simulink model "Impedance_Jawwad"  (R2023a)
settings: Solver=VariableStepAuto  StartTime=0.0  StopTime=10.0  RelTol=1e-3
values from neighbouring files (symbols this model uses):
  Kd = diag([50,50,50,50,50,50])    [parameters.m]
  Kp = diag([250,250,250,250,250,250])    [parameters.m]
  Md = diag([3,3,3,3,3,3])    [parameters.m]
undefined symbols (not defined in the file or in its folder): parms
libraries: robotcorelib x1
settings Model: Creator=uzair  LastModifiedBy=syedj
settings OptimizationCC: ReuseModelBlockBuffer=off

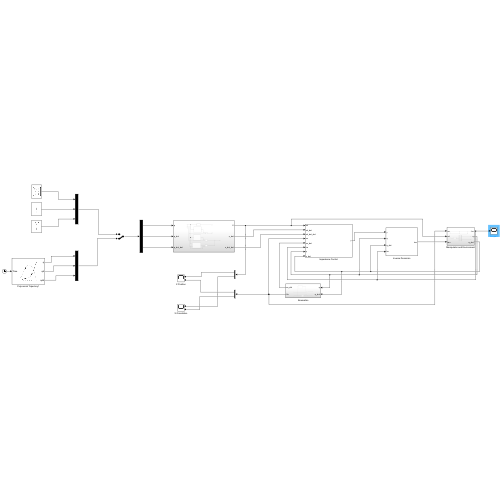
[thumbnail: Simulink's stored preview of the top-level diagram]
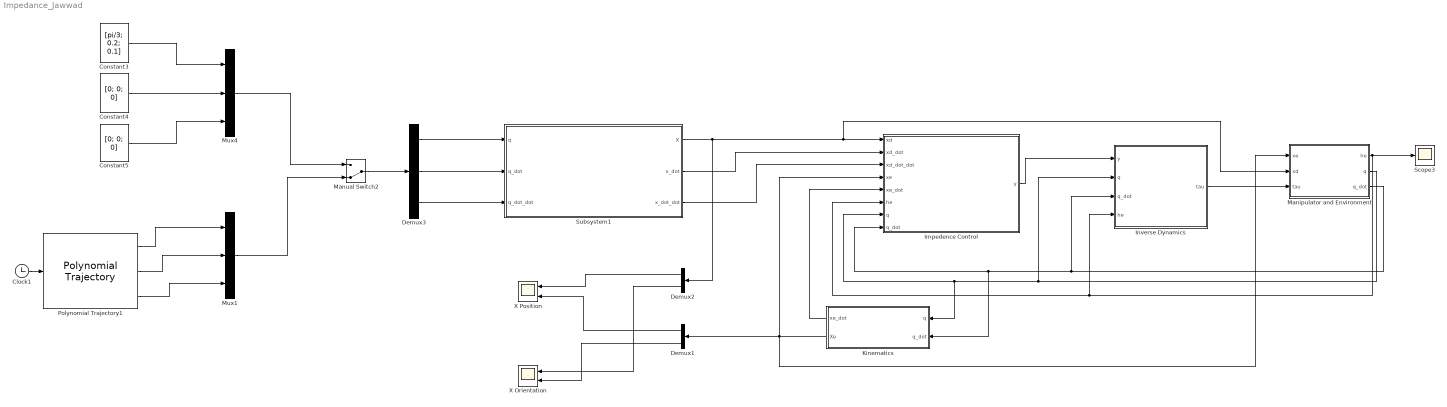
== system Impedance_Jawwad ==
  Clock1 : Clock
  Constant3 : Constant  Value=[pi/3; 0.2; 0.1]  VectorParams1D=off
  Constant4 : Constant  Value=[0; 0; 0]  VectorParams1D=off
  Constant5 : Constant  Value=[0; 0; 0]  VectorParams1D=off
  Demux1 : Demux  Outputs=2
  Demux2 : Demux  Outputs=2
  Demux3 : Demux  Outputs=3
  Impedence Control : Subsystem
  Inverse Dynamics : Subsystem
  Kinematics : Subsystem
  Manipulator and Environment : Subsystem
  Manual Switch2 : ManualSwitch  CurrentSetting=0
  Mux1 : Mux  Inputs=3
  Mux4 : Mux  Inputs=3
  Polynomial Trajectory1 : robotcorelib/Polynomial Trajectory  WaypointSource=Internal  Waypoints=[ 0,0.5,0.7,0.9; 0,-0.05,-0.1,-0.1; 0,0.5,0.7,0.9]  TimePoints=[ 0, 4, 7, 10]  TimeInterval=[ 1, 4 ]  Method=Cubic Polynomial  ParameterSource=Internal  VelocityBoundaryCondition=zeros( 3,4 )  AccelerationBoundaryCondition=zeros( 3,4 )  SimulateUsing=Interpreted execution
  Scope3 : Scope
  Subsystem1 : Subsystem
  X Orientation : Scope  NumInputPorts=2
  X Position : Scope  NumInputPorts=2
  wires:
  Demux1/2 -> X Orientation/2
  Demux2/2 -> X Orientation/1
  Demux2/1 -> X Position/1
  Demux1/1 -> X Position/2
  Manual Switch2/1 -> Demux3/1
  Mux4/1 -> Manual Switch2/1
  Constant4/1 -> Mux4/2
  Polynomial Trajectory1/1 -> Mux1/1
  Polynomial Trajectory1/3 -> Mux1/3
  Mux1/1 -> Manual Switch2/2
  Constant5/1 -> Mux4/3
  Clock1/1 -> Polynomial Trajectory1/1
  Constant3/1 -> Mux4/1
  Demux3/3 -> Subsystem1/3(q_dot_dot)
  Polynomial Trajectory1/2 -> Mux1/2
  Demux3/2 -> Subsystem1/2(q_dot)
  Impedence Control/1(y) -> Inverse Dynamics/1(y)
  Subsystem1/1(X) -> Demux2/1, Manipulator and Environment/2(xd), Impedence Control/1(xd)
  Subsystem1/2(x_dot) -> Impedence Control/2(xd_dot)
  Subsystem1/3(x_dot_dot) -> Impedence Control/3(xd_dot_dot)
  Kinematics/2(Xe) -> Manipulator and Environment/1(xe), Demux1/1, Impedence Control/4(xe)
  Kinematics/1(xe_dot) -> Impedence Control/5(xe_dot)
  Manipulator and Environment/2(q) -> Inverse Dynamics/2(q), Kinematics/1(q), Impedence Control/7(q)
  Manipulator and Environment/3(q_dot) -> Inverse Dynamics/3(q_dot), Kinematics/2(q_dot), Impedence Control/8(q_dot)
  Manipulator and Environment/1(he) -> Scope3/1, Inverse Dynamics/4(he), Impedence Control/6(he)
  Inverse Dynamics/1(tau) -> Manipulator and Environment/3(tau)
  Demux3/1 -> Subsystem1/1(q)

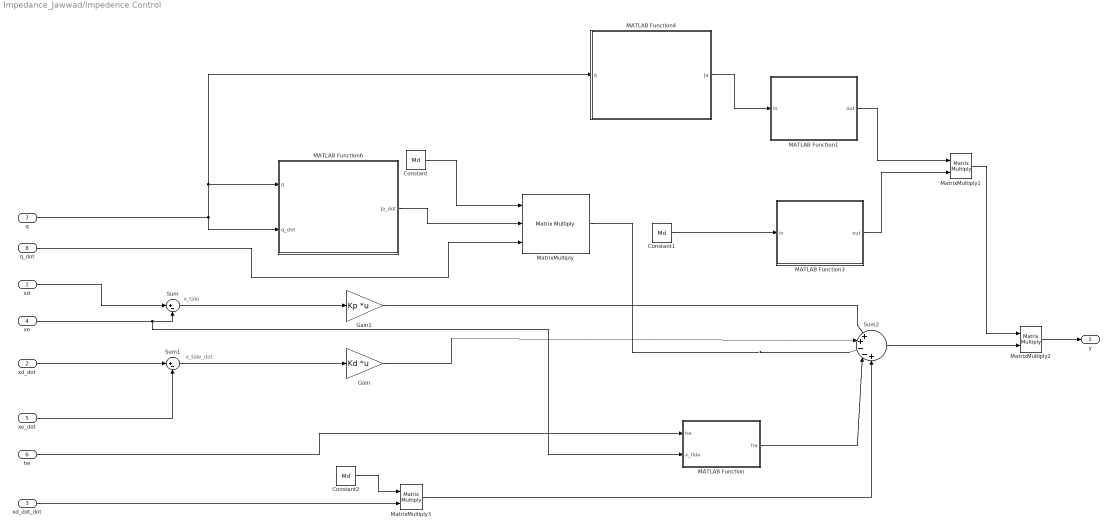
== system Impedance_Jawwad/Impedence Control ==
  note: x_tide_dot
  note: x_tide
  xd : Inport
  xd_dot : Inport  Port=2
  xd_dot_dot : Inport  Port=3
  xe : Inport  Port=4
  xe_dot : Inport  Port=5
  he : Inport  Port=6
  q : Inport  Port=7
  q_dot : Inport  Port=8
  Constant : Constant  Value=Md  VectorParams1D=off
  Constant1 : Constant  Value=Md  VectorParams1D=off
  Constant2 : Constant  Value=Md
  Gain : Gain  Gain=Kd  Multiplication=Matrix(K*u)
  Gain1 : Gain  Gain=Kp  Multiplication=Matrix(K*u)
  MATLAB Function : MATLAB Function  TreatAsAtomicUnit=on
  MATLAB Function1 : MATLAB Function  TreatAsAtomicUnit=on
  MATLAB Function3 : MATLAB Function  TreatAsAtomicUnit=on
  MATLAB Function4 : MATLAB Function  TreatAsAtomicUnit=on
  MATLAB Function6 : MATLAB Function  TreatAsAtomicUnit=on
  MatrixMultiply : Product  Inputs=3  Multiplication=Matrix(*)
  MatrixMultiply1 : Product  Multiplication=Matrix(*)
  MatrixMultiply2 : Product  Multiplication=Matrix(*)
  MatrixMultiply3 : Product  Multiplication=Matrix(*)
  Sum : Sum  Inputs=|+-
  Sum1 : Sum  Inputs=|+-
  Sum2 : Sum  Inputs=|++--+
  y : Outport
  wires:
  xd/1 -> Sum/1
  xe/1 -> MATLAB Function/2(x_tide), Sum/2
  Sum/1 -> Gain1/1
  xd_dot/1 -> Sum1/1
  xe_dot/1 -> Sum1/2
  Sum1/1 -> Gain/1
  Gain1/1 -> Sum2/1
  Gain/1 -> Sum2/2
  q/1 -> MATLAB Function6/2(q_dot), MATLAB Function4/1(q), MATLAB Function6/1(q)
  q_dot/1 -> MatrixMultiply/3
  Constant/1 -> MatrixMultiply/1
  MATLAB Function6/1(Ja_dot) -> MatrixMultiply/2
  MatrixMultiply/1 -> Sum2/3
  he/1 -> MATLAB Function/1(he)
  MATLAB Function/1(ha) -> Sum2/4
  MATLAB Function1/1(out) -> MatrixMultiply1/1
  MATLAB Function3/1(out) -> MatrixMultiply1/2
  MATLAB Function4/1(Ja) -> MATLAB Function1/1(in)
  Constant1/1 -> MATLAB Function3/1(in)
  Sum2/1 -> MatrixMultiply2/2
  MatrixMultiply1/1 -> MatrixMultiply2/1
  MatrixMultiply2/1 -> y/1
  xd_dot_dot/1 -> MatrixMultiply3/2
  Constant2/1 -> MatrixMultiply3/1
  MatrixMultiply3/1 -> Sum2/5

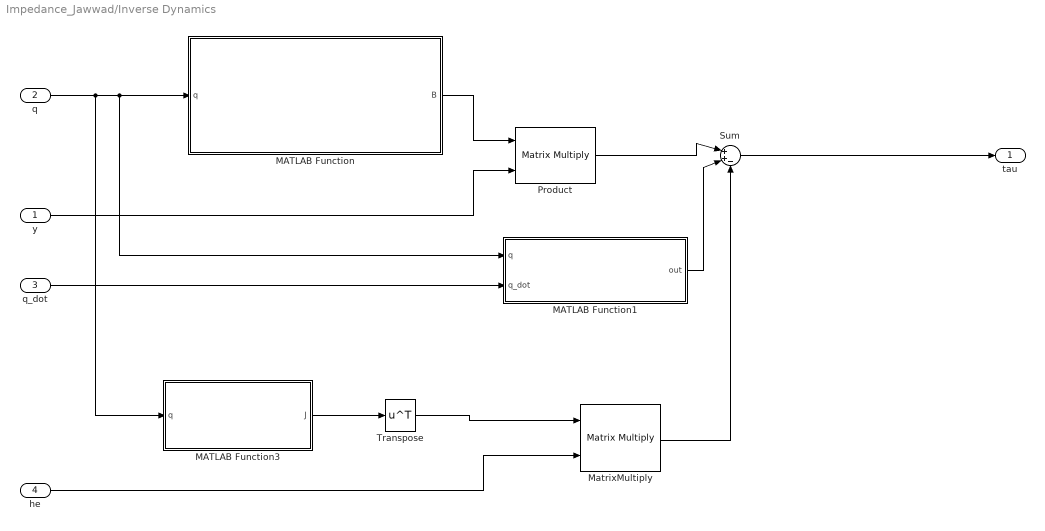
== system Impedance_Jawwad/Inverse Dynamics ==
  y : Inport
  q : Inport  Port=2
  q_dot : Inport  Port=3
  he : Inport  Port=4
  MATLAB Function : MATLAB Function  TreatAsAtomicUnit=on
  MATLAB Function1 : MATLAB Function  TreatAsAtomicUnit=on
  MATLAB Function3 : MATLAB Function  TreatAsAtomicUnit=on
  MatrixMultiply : Product  Multiplication=Matrix(*)
  Product : Product  Multiplication=Matrix(*)
  Sum : Sum  Inputs=|++-
  Transpose : Math  Operator=transpose  OutputSignalType=real
  tau : Outport
  wires:
  q/1 -> MATLAB Function3/1(q), MATLAB Function1/1(q), MATLAB Function/1(q)
  MATLAB Function/1(B) -> Product/1
  y/1 -> Product/2
  q_dot/1 -> MATLAB Function1/2(q_dot)
  MATLAB Function1/1(out) -> Sum/2
  Sum/1 -> tau/1
  MATLAB Function3/1(J) -> Transpose/1
  he/1 -> MatrixMultiply/2
  Transpose/1 -> MatrixMultiply/1
  MatrixMultiply/1 -> Sum/3
  Product/1 -> Sum/1

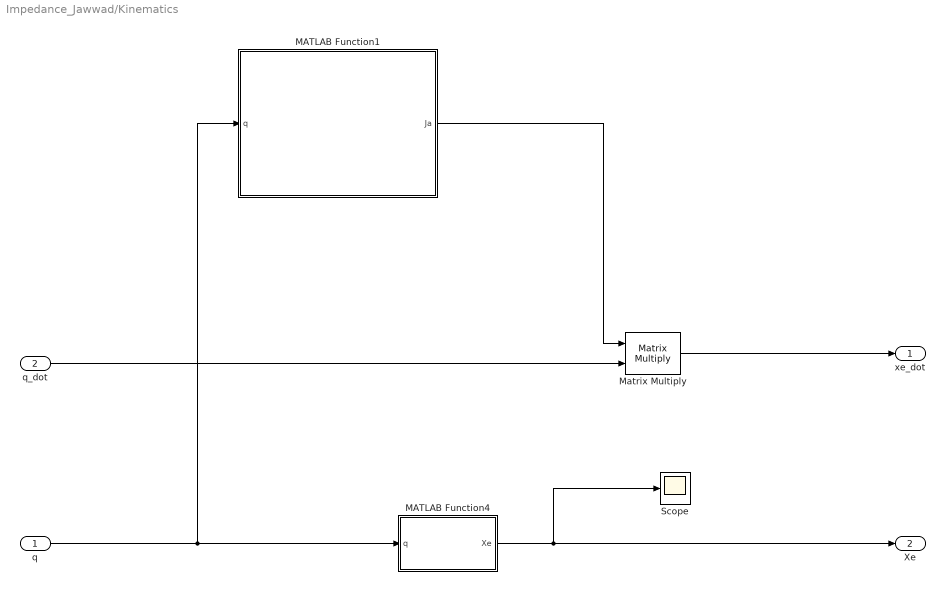
== system Impedance_Jawwad/Kinematics ==
  q : Inport
  q_dot : Inport  Port=2
  MATLAB Function1 : MATLAB Function  TreatAsAtomicUnit=on
  MATLAB Function4 : MATLAB Function  TreatAsAtomicUnit=on
  Matrix Multiply : Product  Multiplication=Matrix(*)
  Scope : Scope
  xe_dot : Outport
  Xe : Outport  Port=2
  wires:
  MATLAB Function1/1(Ja) -> Matrix Multiply/1
  q/1 -> MATLAB Function1/1(q), MATLAB Function4/1(q)
  MATLAB Function4/1(Xe) -> Scope/1, Xe/1
  Matrix Multiply/1 -> xe_dot/1
  q_dot/1 -> Matrix Multiply/2

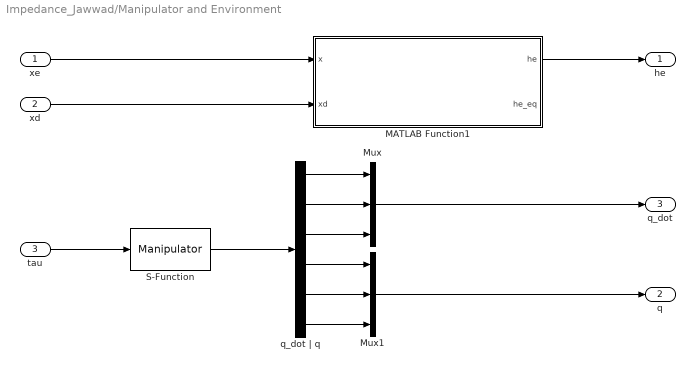
== system Impedance_Jawwad/Manipulator and Environment ==
  xe : Inport
  xd : Inport  Port=2
  tau : Inport  Port=3
  MATLAB Function1 : MATLAB Function  TreatAsAtomicUnit=on
  Mux : Mux  Inputs=3
  Mux1 : Mux  Inputs=3
  S-Function : S-Function  FunctionName=Manipulator  Parameters=params  SFunctionDeploymentMode=off  EnableBusSupport=off
  q_dot | q : Demux  Outputs=6
  he : Outport
  q : Outport  Port=2
  q_dot : Outport  Port=3
  wires:
  xe/1 -> MATLAB Function1/1(x)
  xd/1 -> MATLAB Function1/2(xd)
  MATLAB Function1/1(he) -> he/1
  S-Function/1 -> q_dot | q/1
  q_dot | q/4 -> Mux1/1
  q_dot | q/1 -> Mux/1
  q_dot | q/6 -> Mux1/3
  q_dot | q/2 -> Mux/2
  q_dot | q/5 -> Mux1/2
  q_dot | q/3 -> Mux/3
  Mux/1 -> q_dot/1
  Mux1/1 -> q/1
  tau/1 -> S-Function/1

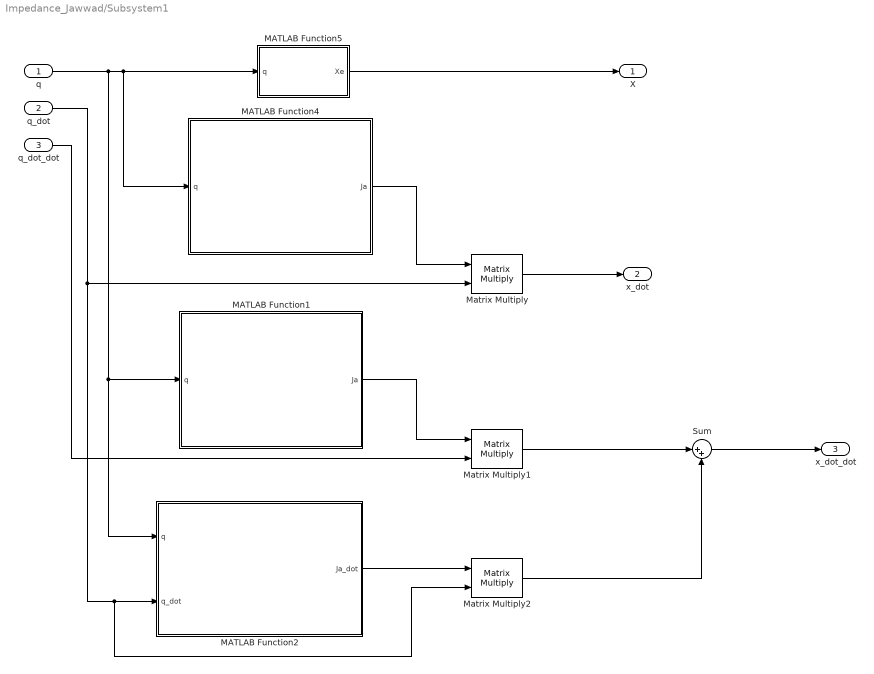
== system Impedance_Jawwad/Subsystem1 ==
  q : Inport
  q_dot : Inport  Port=2
  q_dot_dot : Inport  Port=3
  MATLAB Function1 : MATLAB Function  TreatAsAtomicUnit=on
  MATLAB Function2 : MATLAB Function  TreatAsAtomicUnit=on
  MATLAB Function4 : MATLAB Function  TreatAsAtomicUnit=on
  MATLAB Function5 : MATLAB Function  TreatAsAtomicUnit=on
  Matrix Multiply : Product  Multiplication=Matrix(*)
  Matrix Multiply1 : Product  Multiplication=Matrix(*)  SaturateOnIntegerOverflow=on  LockScale=on
  Matrix Multiply2 : Product  Multiplication=Matrix(*)  InputSameDT=on  SaturateOnIntegerOverflow=on
  Sum : Sum  Inputs=|++
  X : Outport
  x_dot : Outport  Port=2
  x_dot_dot : Outport  Port=3
  wires:
  q/1 -> MATLAB Function2/1(q), MATLAB Function1/1(q), MATLAB Function4/1(q), MATLAB Function5/1(q)
  MATLAB Function5/1(Xe) -> X/1
  Matrix Multiply/1 -> x_dot/1
  q_dot/1 -> MATLAB Function2/2(q_dot), Matrix Multiply2/2, Matrix Multiply/2
  MATLAB Function4/1(Ja) -> Matrix Multiply/1
  MATLAB Function1/1(Ja) -> Matrix Multiply1/1
  q_dot_dot/1 -> Matrix Multiply1/2
  Matrix Multiply1/1 -> Sum/1
  Sum/1 -> x_dot_dot/1
  MATLAB Function2/1(Ja_dot) -> Matrix Multiply2/1
  Matrix Multiply2/1 -> Sum/2

== matlab function Impedance_Jawwad/Impedence Control/MATLAB Function6 ==
  data: q input; Ja_dot output; q_dot input
function Ja_dot = AnalyticalJacobian_Dot(q, q_dot)
q1 = q(1);
q2 = q(2);
q3 = q(3);

q1_dot = q_dot(1);
q2_dot = q_dot(2);
q3_dot = q_dot(3);

    r1 = 0.4;
    a1 = 0.02;
    a2 = 0.03;
    a3 = 0.01;
    b1 = 0.1256;
    b2 = 0.03;
    b3 = 0.01;
    c1 = 0.4;
    c2 = 0.46;
    c3 = 0.15;

     H = [[0, -sin(q1), cos(q1),              cos(q1)*(c1 + c3 + q3)]
[1,        0,       0,                           - c2 - q2]
[0,  cos(q1), sin(q1), r1 + sin(q1)*(c3 + q3) + c1*sin(q1)]
[0,        0,       0,                                   1]];



eulers = rotm2eul(H(1:3,1:3), "ZYZ");


phi1 = eulers(1);
phi2 = eulers(2);
phi3 = eulers(3); %not used

Ja_dot_m = [
[        -cos(q1)*q1_dot*(c1 + c3 + q3)-sin(q1)*q3_dot,  0, -sin(q1)*q1_dot]
[                              0, 0,       0]
[         -sin(q1)*q1_dot*(c1 + c3 + q3)+cos(q1)*q3_dot,  0, cos(q1)*q1_dot]
[(cos(phi2)*sin(phi1))/sin(phi2),  0,       0]
[                     -cos(phi1),  0,       0]
[           -sin(phi1)/sin(phi2),  0,       0]
];

Ja_dot = Ja_dot_m;
end

== matlab function Impedance_Jawwad/Subsystem1/MATLAB Function2 ==
  data: q input; Ja_dot output; q_dot input
function Ja_dot = AnalyticalJacobian_Dot(q, q_dot)
q1 = q(1);
q2 = q(2);
q3 = q(3);

q1_dot = q_dot(1);
q2_dot = q_dot(2);
q3_dot = q_dot(3);

    r1 = 0.4;
    a1 = 0.02;
    a2 = 0.03;
    a3 = 0.01;
    b1 = 0.1256;
    b2 = 0.03;
    b3 = 0.01;
    c1 = 0.4;
    c2 = 0.46;
    c3 = 0.15;

    H = [[0, -sin(q1), cos(q1),              cos(q1)*(c1 + c3 + q3)]
[1,        0,       0,                           - c2 - q2]
[0,  cos(q1), sin(q1), r1 + sin(q1)*(c3 + q3) + c1*sin(q1)]
[0,        0,       0,                                   1]];



eulers = rotm2eul(H(1:3,1:3), "ZYZ");


phi1 = eulers(1);
phi2 = eulers(2);
phi3 = eulers(3); %not used

Ja_dot_m = [
[        -cos(q1)*q1_dot*(c1 + c3 + q3)-sin(q1)*q3_dot,  0, -sin(q1)*q1_dot]
[                              0, 0,       0]
[         -sin(q1)*q1_dot*(c1 + c3 + q3)+cos(q1)*q3_dot,  0, cos(q1)*q1_dot]
[(cos(phi2)*sin(phi1))/sin(phi2),  0,       0]
[                     -cos(phi1),  0,       0]
[           -sin(phi1)/sin(phi2),  0,       0]
];

Ja_dot = Ja_dot_m;
end

== matlab function Impedance_Jawwad/Subsystem1/MATLAB Function4 ==
  data: q input; Ja output
function Ja = AnalyticalJacobian(q)
    q1 = q(1);
    q2 = q(2);
    q3 = q(3);

    r1 = 0.4;
    a1 = 0.02;
    a2 = 0.03;
    a3 = 0.01;
    b1 = 0.1256;
    b2 = 0.03;
    b3 = 0.01;
    c1 = 0.4;
    c2 = 0.46;
    c3 = 0.15;

    H = [[0, -sin(q1), cos(q1),              cos(q1)*(c1 + c3 + q3)]
[1,        0,       0,                           - c2 - q2]
[0,  cos(q1), sin(q1), r1 + sin(q1)*(c3 + q3) + c1*sin(q1)]
[0,        0,       0,                                   1]];


eulers = rotm2eul(H(1:3,1:3), "ZYZ");


    phi1 = eulers(1);
    phi2 = eulers(2);
    phi3 = eulers(3); %not used

Ja_m = [
[        -sin(q1)*(c1 + c3 + q3),  0, cos(q1)]
[                              0, -1,       0]
[         cos(q1)*(c1 + c3 + q3),  0, sin(q1)]
[(cos(phi2)*sin(phi1))/sin(phi2),  0,       0]
[                     -cos(phi1),  0,       0]
[           -sin(phi1)/sin(phi2),  0,       0]
];


    Ja = Ja_m;
end

== matlab function Impedance_Jawwad/Subsystem1/MATLAB Function5 ==
  data: q input; Xe output
function Xe = Kinematics(q)
    q1 = q(1);
    q2 = q(2);
    q3 = q(3);

    r1 = 0.4;
    a1 = 0.02;
    a2 = 0.03;
    a3 = 0.01;
    b1 = 0.1256;
    b2 = 0.03;
    b3 = 0.01;
    c1 = 0.4;
    c2 = 0.46;
    c3 = 0.15;

    H = [[0, -sin(q1), cos(q1),              cos(q1)*(c1 + c3 + q3)]
[1,        0,       0,                           - c2 - q2]
[0,  cos(q1), sin(q1), r1 + sin(q1)*(c3 + q3) + c1*sin(q1)]
[0,        0,       0,                                   1]];

    eulers = rotm2eul(H(1:3,1:3), "ZYZ");

    Xe = [H(1:3,4); eulers'];
end

== matlab function Impedance_Jawwad/Inverse Dynamics/MATLAB Function1 ==
  data: q input; out output; q_dot input; params parameter
function out = n(q, q_dot, params)
    
    m1 = params.m(1);
    m2 = params.m(2);
    m3 = params.m(3);

    q1 = q(1);
    q2 = q(2);
    q3 = q(3);

    q1_dot = q_dot(1);
    q2_dot = q_dot(2);
    q3_dot = q_dot(3);
    
    r1 = 0.4;
    a1 = 0.02;
    a2 = 0.03;
    a3 = 0.01;
    b1 = 0.1256;
    b2 = 0.03;
    b3 = 0.01;
    c1 = 0.4;
    c2 = 0.46;
    c3 = 0.15;
    g = params.g;

    Fv = params.Fv;
 

   C = [[ (m3*q3_dot*(2*c1 + c3 + 2*q3))/2, 0, (m3*q1_dot*(2*c1 + c3 + 2*q3))/2]
[                                0, 0,                                0]
[-(m3*q1_dot*(2*c1 + c3 + 2*q3))/2, 0,                                0]];
   

G = [(c1*g*m1*cos(q1))/2 + g*m2*cos(q1)*(c1 - c2/2) + g*m3*cos(q1)*(c1 + c3/2 + q3)
        0;
        g*m3*sin(q1)];

    out = C*q_dot + diag(Fv)*q_dot + G;
end

== matlab function Impedance_Jawwad/Inverse Dynamics/MATLAB Function ==
  data: q input; B output; params parameter
function B = inertiaMatrix(q, params)
    q1 = q(1); % not used in this matrix
    q2 = q(2);
    q3 = q(3);

    m1 = params.m(1);
    m2 = params.m(2);
    m3 = params.m(3);
        
    r1 = 0.4;
    a1 = 0.02;
    a2 = 0.03;
    a3 = 0.01;
    b1 = 0.1256;
    b2 = 0.03;
    b3 = 0.01;
    c1 = 0.4;
    c2 = 0.46;
    c3 = 0.15;

  B = [[(a2^2*m2)/12 + (3*a1^4*m1)/2 + (a3^2*m3)/12 + (3*b1^4*m1)/2 + (b3^2*m3)/12 + c1^2*m1 + c1^2*m2 + c1^2*m3 + (7*c2^2*m2)/12 + (c3^2*m3)/2 + m3*q3^2 + 3*a1^2*b1^2*m1 - c1*c2*m2 + c1*c3*m3 + 2*c1*m3*q3 + c3*m3*q3,       0,  0]
[                                                                                                                                                                                                               0, m2 + m3,  0]
[                                                                                                                                                                                                               0,       0, m3]];
 end

== matlab function Impedance_Jawwad/Subsystem1/MATLAB Function1 ==
  data: q input; Ja output
function Ja = AnalyticalJacobian(q)
    q1 = q(1);
    q2 = q(2);
    q3 = q(3);

    r1 = 0.4;
    a1 = 0.02;
    a2 = 0.03;
    a3 = 0.01;
    b1 = 0.1256;
    b2 = 0.03;
    b3 = 0.01;
    c1 = 0.4;
    c2 = 0.46;
    c3 = 0.15;

    H = [[0, -sin(q1), cos(q1),              cos(q1)*(c1 + c3 + q3)]
[1,        0,       0,                           - c2 - q2]
[0,  cos(q1), sin(q1), r1 + sin(q1)*(c3 + q3) + c1*sin(q1)]
[0,        0,       0,                                   1]];


eulers = rotm2eul(H(1:3,1:3), "ZYZ");


    phi1 = eulers(1);
    phi2 = eulers(2);
    phi3 = eulers(3); %not used

Ja_m = [
[        -sin(q1)*(c1 + c3 + q3),  0, cos(q1)]
[                              0, -1,       0]
[         cos(q1)*(c1 + c3 + q3),  0, sin(q1)]
[(cos(phi2)*sin(phi1))/sin(phi2),  0,       0]
[                     -cos(phi1),  0,       0]
[           -sin(phi1)/sin(phi2),  0,       0]
];


    Ja = Ja_m;
end

== matlab function Impedance_Jawwad/Impedence Control/MATLAB Function ==
  data: he input; ha output; x_tide input
function ha = he_d_e(he, x_tide)

        euler = x_tide(4:6);

        phi1 = euler(1);
        phi2 = euler(2);

        T = [[0, -sin(phi1) ,    cos(phi1)*sin(phi2)];
                 [0,  cos(phi1) ,   sin(phi1)*sin(phi2)];
                 [1,               0  ,    cos(phi2)]];

        Ta = [[eye(3), zeros(3)];
              [zeros(3), T]];


        ha = Ta'*he;
end

== matlab function Impedance_Jawwad/Kinematics/MATLAB Function4 ==
  data: q input; Xe output
function Xe = Kinematics(q)
    q1 = q(1);
    q2 = q(2);
    q3 = q(3);
    
    r1 = 0.4;
    a1 = 0.02;
    a2 = 0.03;
    a3 = 0.01;
    b1 = 0.1256;
    b2 = 0.03;
    b3 = 0.01;
    c1 = 0.4;
    c2 = 0.46;
    c3 = 0.15;


    H = [[0, -sin(q1), cos(q1),              cos(q1)*(c1 + c3 + q3)]
[1,        0,       0,                           - c2 - q2]
[0,  cos(q1), sin(q1), r1 + sin(q1)*(c3 + q3) + c1*sin(q1)]
[0,        0,       0,                                   1]];
    
    eulers = rotm2eul(H(1:3,1:3), "ZYZ");

    Xe = [H(1:3,4); eulers'];
end

== matlab function Impedance_Jawwad/Impedence Control/MATLAB Function1 ==
  data: in input; out output
function out = inv(in)
    out = pinv(in);
end

== matlab function Impedance_Jawwad/Kinematics/MATLAB Function1 ==
  data: q input; Ja output
function Ja = AnalyticalJacobian(q)
    q1 = q(1);
    q2 = q(2);
    q3 = q(3);
    
    r1 = 0.4;
    a1 = 0.02;
    a2 = 0.03;
    a3 = 0.01;
    b1 = 0.1256;
    b2 = 0.03;
    b3 = 0.01;
    c1 = 0.4;
    c2 = 0.46;
    c3 = 0.15;

    H = [[0, -sin(q1), cos(q1),              cos(q1)*(c1 + c3 + q3)]
[1,        0,       0,                           - c2 - q2]
[0,  cos(q1), sin(q1), r1 + sin(q1)*(c3 + q3) + c1*sin(q1)]
[0,        0,       0,                                   1]];


eulers = rotm2eul(H(1:3,1:3), "ZYZ");


    phi1 = eulers(1);
    phi2 = eulers(2);
    phi3 = eulers(3); %not used

Ja_m = [
[        -sin(q1)*(c1 + c3 + q3),  0, cos(q1)]
[                              0, -1,       0]
[         cos(q1)*(c1 + c3 + q3),  0, sin(q1)]
[(cos(phi2)*sin(phi1))/sin(phi2),  0,       0]
[                     -cos(phi1),  0,       0]
[           -sin(phi1)/sin(phi2),  0,       0]
];


    Ja = Ja_m;
end

== matlab function Impedance_Jawwad/Manipulator and Environment/MATLAB Function1 ==
  data: x input; he output; xd input; parms parameter; Kp parameter; he_eq output
function [he,he_eq]= Environment(x, xd, parms, Kp)
    if(x(parms.plane_axis) >= parms.plane_pos(parms.plane_axis))
        xr = parms.plane_pos;

        xdes = zeros(6,1);
        xdes(parms.plane_axis) = xd(parms.plane_axis);

        xe = zeros(6,1);
        xe(parms.plane_axis) = x(parms.plane_axis);

        he = parms.Ke * (xe - xr);

        he_eq = pinv(eye(6) + parms.Ke*pinv(Kp))*parms.Ke*(xdes - xr);

    else
        he = zeros(6,1);
        he_eq = zeros(6,1);
    end
end

== matlab function Impedance_Jawwad/Impedence Control/MATLAB Function3 ==
  data: in input; out output
function out = inv(in)
    out = pinv(in);
end

== matlab function Impedance_Jawwad/Impedence Control/MATLAB Function4 ==
  data: q input; Ja output
function Ja = AnalyticalJacobian(q)
    q1 = q(1);
    q2 = q(2);
    q3 = q(3);
    
    r1 = 0.4;
    a1 = 0.02;
    a2 = 0.03;
    a3 = 0.01;
    b1 = 0.1256;
    b2 = 0.03;
    b3 = 0.01;
    c1 = 0.4;
    c2 = 0.46;
    c3 = 0.15;

    H = [[0, -sin(q1), cos(q1),              cos(q1)*(c1 + c3 + q3)]
[1,        0,       0,                           - c2 - q2]
[0,  cos(q1), sin(q1), r1 + sin(q1)*(c3 + q3) + c1*sin(q1)]
[0,        0,       0,                                   1]];


eulers = rotm2eul(H(1:3,1:3), "ZYZ");


    phi1 = eulers(1);
    phi2 = eulers(2);
    phi3 = eulers(3); %not used

Ja_m = [
[        -sin(q1)*(c1 + c3 + q3),  0, cos(q1)]
[                              0, -1,       0]
[         cos(q1)*(c1 + c3 + q3),  0, sin(q1)]
[(cos(phi2)*sin(phi1))/sin(phi2),  0,       0]
[                     -cos(phi1),  0,       0]
[           -sin(phi1)/sin(phi2),  0,       0]
];


    Ja = Ja_m;
end

== matlab function Impedance_Jawwad/Inverse Dynamics/MATLAB Function3 ==
  data: q input; J output
function J = GeomatricalJacobian(q)
q1 = q(1);
q2 = q(2);
q3 = q(3);
    
    r1 = 0.4;
    a1 = 0.02;
    a2 = 0.03;
    a3 = 0.01;
    b1 = 0.1256;
    b2 = 0.03;
    b3 = 0.01;
    c1 = 0.4;
    c2 = 0.46;
    c3 = 0.15;

    J = [
[-sin(q1)*(c1 + c3 + q3),  0, cos(q1)]
[                      0, -1,       0]
[ cos(q1)*(c1 + c3 + q3),  0, sin(q1)]
[                      0,  0,       0]
[                     -1,  0,       0]
[                      0,  0,       0]];

end
